simulink model "LeadLagSimulation"  (R2024b)
settings: Solver=VariableStepAuto  StartTime=0.0  StopTime=10.0  RelTol=1e-5
values from neighbouring files (symbols this model uses):
  omega = 78    [LeadLagController.m]
settings Model: Creator=mahmo  LastModifiedBy=mahmo

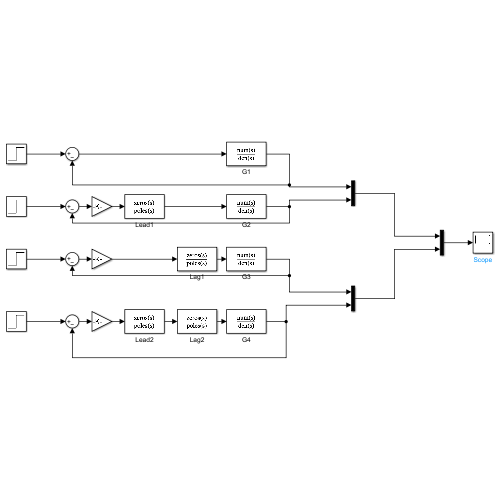
[thumbnail: Simulink's stored preview of the top-level diagram]
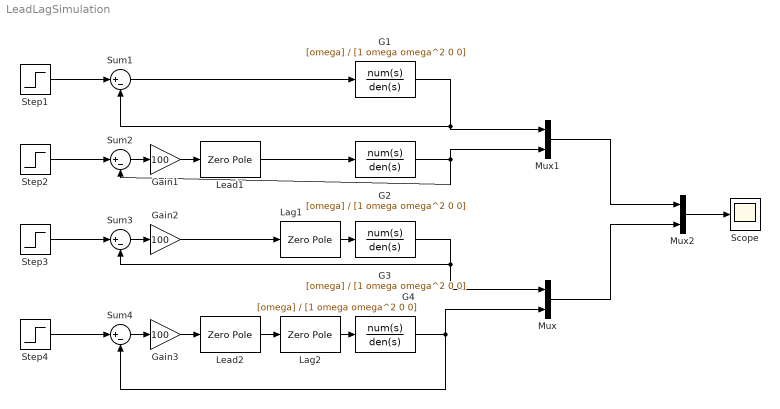
== system LeadLagSimulation ==
  G{1..4} (4 alike) : TransferFcn  Numerator=[omega]  Denominator=[1 omega omega^2 0 0]
  Gain1 : Gain  Gain=100
  Gain2 : Gain  Gain=100
  Gain3 : Gain  Gain=100
  Lag1 : ZeroPole  Zeros=[-0.1]  Poles=[-0.02]  ContinuousStateAttributes='Lag'
  Lag2 : ZeroPole  Zeros=[-0.1]  Poles=[-0.002]  ContinuousStateAttributes='Lag'
  Lead1 : ZeroPole  Zeros=[-0.25]  Poles=[-2]  ContinuousStateAttributes='Lead'
  Lead2 : ZeroPole  Zeros=[-0.25]  Poles=[-2]  ContinuousStateAttributes='Lead'
  Mux : Mux  Inputs=2
  Mux1 : Mux  Inputs=2
  Mux2 : Mux  Inputs=2
  Scope : Scope
  Step{1..4} (4 alike) : Step  SampleTime=0
  Sum{1..4} (4 alike) : Sum  Inputs=|+-
  wires:
  Gain3/1 -> Lead2/1
  Step4/1 -> Sum4/1
  Lead2/1 -> Lag2/1
  Sum4/1 -> Gain3/1
  G4/1 -> Mux/2, Sum4/2
  Lag2/1 -> G4/1
  G1/1 -> Mux1/1, Sum1/2
  Step1/1 -> Sum1/1
  Sum1/1 -> G1/1
  Step2/1 -> Sum2/1
  Gain1/1 -> Lead1/1
  Lead1/1 -> G2/1
  Sum2/1 -> Gain1/1
  G2/1 -> Mux1/2, Sum2/2
  Sum3/1 -> Gain2/1
  Lag1/1 -> G3/1
  Gain2/1 -> Lag1/1
  G3/1 -> Mux/1, Sum3/2
  Step3/1 -> Sum3/1
  Mux1/1 -> Mux2/1
  Mux/1 -> Mux2/2
  Mux2/1 -> Scope/1
